simulink model "wirkungsplan_mdl"  (R2013b)
settings: Solver=ode45  StartTime=0.0  StopTime=10.0  RelTol=1e-3
values from neighbouring files (symbols this model uses):
  a = 0.001    [wirkungsplan.m]
  J = 0.00025    [wirkungsplan.m]
  K = 0.05    [wirkungsplan.m]
  R = 0.5    [wirkungsplan.m]
settings Model: Creator=daniw  LastModifiedBy=daniw

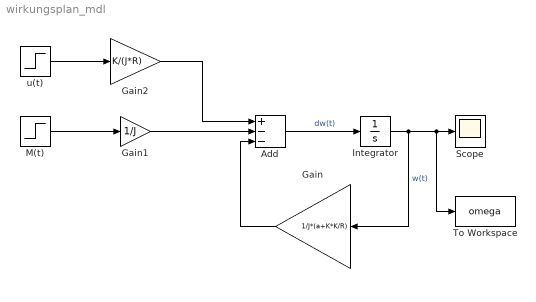
== system wirkungsplan_mdl ==
  Add : Sum  Inputs=+--
  Gain : Gain  Gain=1/J*(a+K*K/R)
  Gain1 : Gain  Gain=1/J
  Gain2 : Gain  Gain=K/(J*R)
  Integrator : Integrator
  M(t) : Step  Time=2  SampleTime=0
  Scope : Scope
  To Workspace : ToWorkspace  VariableName=omega  SampleTime=-1  SaveFormat=Structure With Time
  u(t) : Step  Before=5  After=20  SampleTime=0
  wires:
  Add/1 -> Integrator/1  "dw(t)"
  Integrator/1 -> To Workspace/1, Scope/1, Gain/1  "w(t)"
  Gain/1 -> Add/3
  M(t)/1 -> Gain1/1
  Gain1/1 -> Add/2
  u(t)/1 -> Gain2/1
  Gain2/1 -> Add/1
